simulink model "Stabilization_simulink"  (R2025b)
settings: Solver=ode4  StartTime=0.0  StopTime=1  FixedStep=1/200  RelTol=1e-3
undefined symbols (not defined in the file or in its folder): dz, input_deg, Ki, Km, Kp, Pm, W_sat, wb_dist
settings Model: Creator=chaeeun  LastModifiedBy=ADMIN

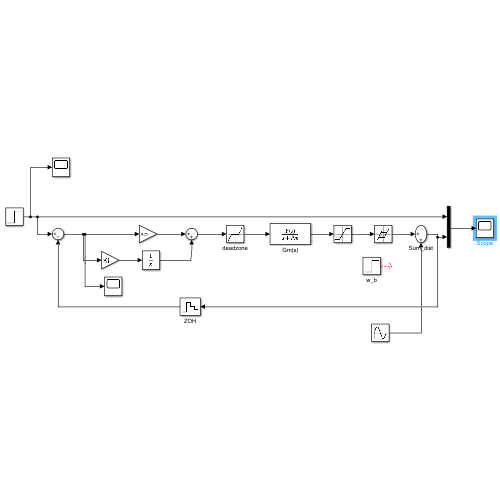
[thumbnail: Simulink's stored preview of the top-level diagram]
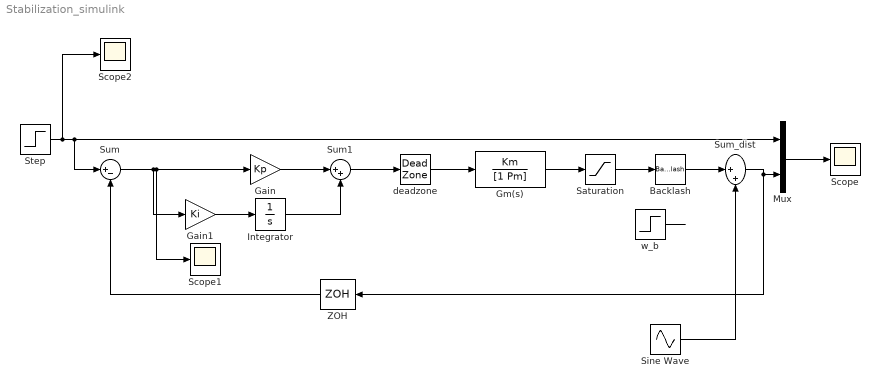
== system Stabilization_simulink ==
  Backlash : Backlash  BacklashWidth=3
  Gain : Gain  Gain=Kp
  Gain1 : Gain  Gain=Ki
  Gm(s) : TransferFcn  Numerator=Km  Denominator=[1 Pm]
  Integrator : Integrator
  Mux : Mux  Inputs=2
  Saturation : Saturate  UpperLimit=W_sat  LowerLimit=-W_sat
  Scope : Scope
      settings: ActiveDisplayYMinimum=-2.8795728821502262  ActiveDisplayYMaximum=9.6135208856703454
  Scope1 : Scope
      settings: ActiveDisplayYMinimum=-1  ActiveDisplayYMaximum=1
  Scope2 : Scope
      settings: ActiveDisplayYMinimum=-1  ActiveDisplayYMaximum=1  DataLoggingVariableName=ScopeData2
  Sine Wave : Sin  Frequency=0.5*2*pi  SampleTime=0
  Step : Step  Time=0  After=input_deg  SampleTime=0  VectorParams1D=off
  Sum : Sum  Inputs=|+-
  Sum1 : Sum  Inputs=|++
  Sum_dist : Sum  Inputs=|++
  ZOH : ZeroOrderHold  SampleTime=1/200
  deadzone : DeadZone  LowerValue=-dz  UpperValue=dz
  w_b : Step  Time=0.25  After=wb_dist  SampleTime=0  VectorParams1D=off
  wires:
  ZOH/1 -> Sum/2
  Mux/1 -> Scope/1
  Sum_dist/1 -> ZOH/1, Mux/2
  Step/1 -> Scope2/1, Mux/1, Sum/1
  Gain/1 -> Sum1/1
  Sum/1 -> Gain/1, Scope1/1, Gain1/1
  Gain1/1 -> Integrator/1
  Integrator/1 -> Sum1/2
  Sum1/1 -> deadzone/1
  deadzone/1 -> Gm(s)/1
  Gm(s)/1 -> Saturation/1
  Saturation/1 -> Backlash/1
  Backlash/1 -> Sum_dist/1
  w_b/1 -> ?
  Sine Wave/1 -> Sum_dist/2
